simulink model "differential_drive"  (R2018a)
settings: Solver=FixedStepAuto  StartTime=0.0  StopTime=20  FixedStep=0.01  RelTol=1e-3
settings Model: EnablePacing=on  Creator=U500304  LastModifiedBy=U500304
settings SolverCC: ZeroCrossAlgorithm=Adaptive
settings DataIOCC: SaveOutput=off  SaveTime=off
settings DebuggingCC: MaxConsecutiveZCsMsg=none

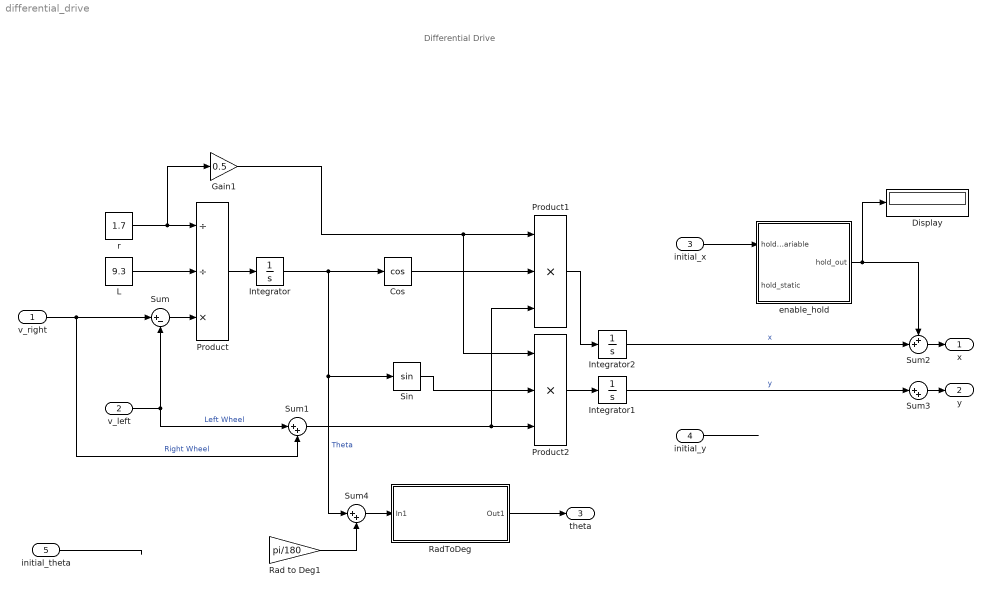
== system differential_drive ==
  note: Differential Drive
  v_right : Inport  OutDataTypeStr=double  PortDimensions=1
  v_left : Inport  Port=2  OutDataTypeStr=double  PortDimensions=1
  initial_x : Inport  Port=3
  initial_y : Inport  Port=4
  initial_theta : Inport  Port=5
  Cos : Trigonometry  Operator=cos
  Display : Display
  Gain1 : Gain  Gain=0.5
  Integrator : Integrator
  Integrator1 : Integrator
  Integrator2 : Integrator
  L : Constant  Value=9.3
  Product : Product  Inputs=//*
  Product1 : Product  Inputs=3
  Product2 : Product  Inputs=3
  Rad to Deg1 : Gain  Gain=pi/180
  RadToDeg : Subsystem
  Sin : Trigonometry
  Sum : Sum  Inputs=|+-
  Sum1 : Sum  Inputs=|++
  Sum2 : Sum  Inputs=++|
  Sum3 : Sum  Inputs=|++
  Sum4 : Sum  Inputs=|++
  enable_hold : Subsystem
  r : Constant  Value=1.7
  x : Outport  OutDataTypeStr=double  PortDimensions=1  SampleTime=0
  y : Outport  Port=2  OutDataTypeStr=double  PortDimensions=1  SampleTime=0
  theta : Outport  Port=3  OutDataTypeStr=double  PortDimensions=1  SampleTime=0
  wires:
  v_right/1 -> Sum/1, Sum1/2  "Right Wheel"
  L/1 -> Product/2
  Sum1/1 -> Product2/3, Product1/3
  r/1 -> Product/1, Gain1/1
  Gain1/1 -> Product2/1, Product1/1
  Sin/1 -> Product2/2
  v_left/1 -> Sum1/1, Sum/2  "Left Wheel"
  Integrator/1 -> Cos/1, Sum4/1, Sin/1  "Theta"
  Product/1 -> Integrator/1
  Product2/1 -> Integrator1/1
  Cos/1 -> Product1/2
  Sum/1 -> Product/3
  Product1/1 -> Integrator2/1
  Integrator1/1 -> Sum3/1  "y"
  Sum2/1 -> x/1
  initial_x/1 -> enable_hold/1(hold_variable)
  Sum3/1 -> y/1
  initial_y/1 -> ?
  initial_theta/1 -> ?
  Rad to Deg1/1 -> Sum4/2
  Sum4/1 -> RadToDeg/1(In1)
  RadToDeg/1(Out1) -> theta/1
  Integrator2/1 -> Sum2/2  "x"
  enable_hold/1(hold_out) -> Display/1, Sum2/1
  ? -> Sum3/2

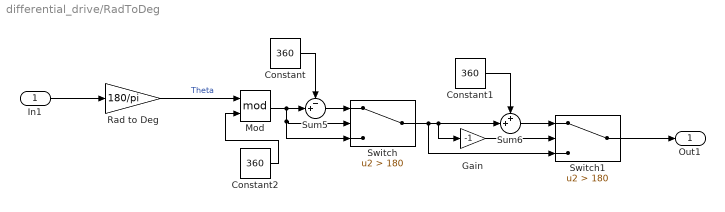
== system differential_drive/RadToDeg ==
  In1 : Inport
  Constant : Constant  Value=360
  Constant1 : Constant  Value=360
  Constant2 : Constant  Value=360
  Gain : Gain  Gain=-1
  Mod : Math  Operator=mod  SaturateOnIntegerOverflow=on
  Rad to Deg : Gain  Gain=180/pi
  Sum5 : Sum  Inputs=-+|
  Sum6 : Sum  Inputs=++|
  Switch : Switch  Criteria=u2 > Threshold  Threshold=180
  Switch1 : Switch  Criteria=u2 > Threshold  Threshold=180
  Out1 : Outport
  wires:
  Constant/1 -> Sum5/1
  Constant1/1 -> Sum6/1
  Rad to Deg/1 -> Mod/1  "Theta"
  Gain/1 -> Switch1/2
  Switch/1 -> Sum6/2, Gain/1, Switch1/3
  Sum5/1 -> Switch/1
  Mod/1 -> Sum5/2, Switch/2, Switch/3
  Sum6/1 -> Switch1/1
  Constant2/1 -> Mod/2
  In1/1 -> Rad to Deg/1
  Switch1/1 -> Out1/1

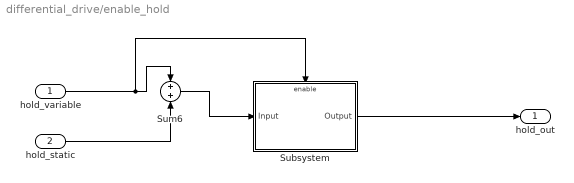
== system differential_drive/enable_hold ==
  hold_variable : Inport
  hold_static : Inport  Port=2
  Subsystem : Subsystem
  Sum6 : Sum
  hold_out : Outport
  wires:
  Sum6/1 -> Subsystem/1(Input)
  Subsystem/1(Output) -> hold_out/1
  hold_static/1 -> Sum6/2
  hold_variable/1 -> Sum6/1, Subsystem/Enable

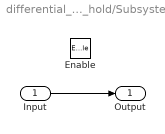
== system differential_drive/enable_hold/Subsystem ==
  Input : Inport
  Enable : EnablePort
  Output : Outport
  wires:
  Input/1 -> Output/1
